simulink model "SMC_linear_c"  (R2015b)
settings: Solver=VariableStepAuto  StartTime=0.0  StopTime=10.0  RelTol=1e-3
undefined symbols (not defined in the file): Asmc, Bsmc, mu, p
settings Model: Creator=mgreiff  LastModifiedBy=mgreiff

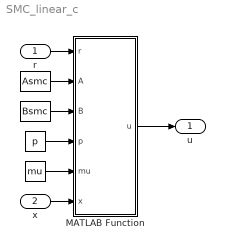
== system SMC_linear_c ==
  r : Inport  PortDimensions=3
  x : Inport  Port=2  PortDimensions=3
  "     " : Constant  Value=Asmc
  "      " : Constant  Value=Bsmc
  "        " : Constant  Value=p
  "         " : Constant  Value=mu
  MATLAB Function : MATLAB Function  TreatAsAtomicUnit=on
  u : Outport
  wires:
  r/1 -> MATLAB Function/1(r)
  "     "/1 -> MATLAB Function/2(A)
  "      "/1 -> MATLAB Function/3(B)
  "        "/1 -> MATLAB Function/4(p)
  "         "/1 -> MATLAB Function/5(mu)
  MATLAB Function/1(u) -> u/1
  x/1 -> MATLAB Function/6(x)

== matlab function SMC_linear_c/MATLAB Function ==
  data: r input; A input; B input; p input; mu input; u output; x input
function u = SMC(r, A, B, p, mu, x)
%#codegen
e = x - r;
u = -((p' * A * x)/(p' * B)) - (mu/(p' * B)) * sign(p'*e);
